simulink model "MarkImage"  (R2019a)
settings: Solver=VariableStepAuto  StartTime=0.0  StopTime=10.0  RelTol=1e-3
libraries: embdlinuxlib x1
settings Model: Creator=wojna  LastModifiedBy=wojna

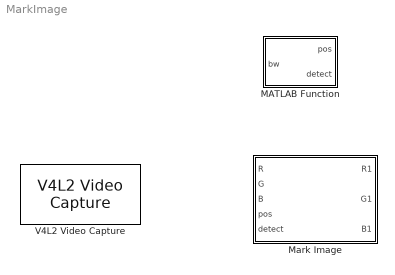
== system MarkImage ==
  MATLAB Function : MATLAB Function  TreatAsAtomicUnit=on
  "Mark Image " : MATLAB Function  TreatAsAtomicUnit=on
  V4L2 Video Capture : embdlinuxlib/V4L2 Video Capture  m_devName='/dev/video0'  roi=[0, 0, 640, 480]  imSizeSelection=160x120  imSize=[640, 480]  pixelFormat=RGB  pixelOrder=Planar  sampleTime=0.05  simOutput=Colorbars  blockPlatform=Raspberry Pi
      settings: SourceProductName=Simulink Coder Support Package for BeagleBone Blue Hardware  SourceProductBaseCode=SC_BEAGLEBONE_BLUE

== matlab function MarkImage/MATLAB Function ==
  data: bw input; pos output; detect output
function [pos, detect] = FindCentroid(bw)

[r,c]=find(bw);
if isempty(r)
    pos = [-1 -1];
    detect = false;
else
    pos = [mean(r), mean(c)];
    detect = true;
end

== matlab function MarkImage/Mark Image  ==
  data: R input; R1 output; G input; B input; pos input; detect input; G1 output; B1 output
function [R1,G1,B1] = MarkImage(R,G,B, pos, detect)
R1 = R; G1 = G; B1 = B;
if detect
    R1(pos(1)-3:pos(1)+3, pos(2)-3:pos(2)+3) = 255;
    G1(pos(1)-3:pos(1)+3, pos(2)-3:pos(2)+3) = 0; 
    B1(pos(1)-3:pos(1)+3, pos(2)-3:pos(2)+3) = 0;
end
